simulink model "flightControlSystem"  (R2025b)
settings: Solver=ode3  StartTime=0  StopTime=TFinal  FixedStep=Ts  RelTol=1e-3  EnableMultiTasking=on
undefined symbols (not defined in the file): codertarget, Controller, DiscIntNeverNeededParam, Discrete, Estimator, g, gray, init, orient_ref, pos_ref, Sensors, Time, Ts, var_acc_angle_N, var_bias_gyr_N, var_gyro_p_N, Vehicle
libraries: simulink x40, slpidlib x5, ctrlSharedLib x4, sharedtransform x3, visiontextngfix x1, parrotlib x1
(part 3 of 3)

== matlab function flightControlSystem/Image Processing System/MATLAB Function ==
  data: var_yok input; binaryImg input; line_coords output; line_colors output; yaw_angle output; current_yaw input; length_90 output; on_track output; land_now output; detected output; target_offset output
function [line_coords, line_colors, yaw_angle, length_90, on_track,land_now,detected,target_offset] = pathFollower(var_yok, binaryImg, current_yaw)
% --- PARAMETRELER VE MATRİS HAZIRLIĞI ---
H = 90; W = 60; 
x0 = 30; y0 = 60;
angles = -15:5:195; % Bu 41 elemanlı bir dizidir
numAngles = length(angles); % Dinamik olarak 37 olur
maxLen = 200;
coder.extrinsic('imfindcircles');

% Matris boyutlarını 37 ışın + 2 güvenlik noktası = 39 yapıyoruz
line_coords = zeros(46,4);
line_colors = zeros(46,3); 

% Başlangıçta tüm çizgileri yeşil yap
for i = 1:45
    line_colors(i,:) = [0 250 0];
end

lengths = zeros(numAngles, 1);
on_track = 1; 

% --- 1. IŞINSAL (RAY-CASTING) TARAMA ---
for i = 1:numAngles
    theta = angles(i) * pi/180;
    r = 0;
    for k = 1:maxLen
        x = round(x0 + k*cos(theta));
        y = round(y0 - k*sin(theta));
        
        if x < 1 || x > W || y < 1 || y > H || binaryImg(y,x) == 0
            break;
        end
        r = k;
    end
    x_end = round(x0 + r*cos(theta));
    y_end = round(y0 - r*sin(theta));
    
    line_coords(i,:) = [x0 y0 x_end y_end];
    lengths(i) = r;
end

% Sağ (1. ışın) ve Sol (Sonuncu ışın) çizgilerini MOR yap
line_colors(1, :) = [160 32 240];   % Mor (Purple)
line_colors(numAngles, :) = [160 32 240]; 

% --- DİĞER HESAPLAMALAR ---
% En uzun 3 çizgiyi bul ve kırmızı yap (Eğer morlarla çakışmazsa)
[~, idx] = sort(lengths, 'descend');
top_idxs = idx(1:3);
for j = 1:3
    % Eğer en uzunlardan biri 0 veya 180 değilse kırmızı yap
    if top_idxs(j) ~= 1 && top_idxs(j) ~= numAngles
        line_colors(top_idxs(j), :) = [245 0 0];
    end
end

% 90 derece (Tam ön - 19. eleman) çizgisini mavi yap
line_colors(22, :) = [0 0 255]; 
length_90 = lengths(22);

% --- 2. GÜVENLİK KOLLARI VE ON_TRACK KONTROLÜ ---
offset_x = 6; offset_y = 18; 
right_x = max(1, min(W, round(x0 + offset_x)));
left_x  = max(1, min(W, round(x0 - offset_x)));
check_y = max(1, min(H, round(y0 - offset_y)));

if binaryImg(check_y, right_x) == 0 || binaryImg(check_y, left_x) == 0
    on_track = 0; 
end

% --- 3. YAW HESAPLAMA ---
if var_yok == 1
        w1 = lengths(top_idxs(1)); w2 = lengths(top_idxs(2)); w3 = lengths(top_idxs(3));
        avg_angle_deg = (angles(top_idxs(1))*w1 + angles(top_idxs(2))*w2 + angles(top_idxs(3))*w3) / (w1 + w2 + w3);
        error_yaw = (avg_angle_deg - 90) * pi/180;
        yaw_angle = current_yaw + (error_yaw);
else
    yaw_angle = current_yaw;
end

% --- 4. GÖRSELLEŞTİRME (38. ve 39. SATIRLAR) ---
line_coords(44,:) = [right_x, check_y, right_x+1, check_y];
line_coords(45,:) = [left_x, check_y, left_x+1, check_y];

% Güvenlik noktaları renkleri
if binaryImg(check_y, right_x) == 0
    line_colors(44,:) = [0 0 0]; 
else
    line_colors(44,:) = [255 255 255]; 
end

if binaryImg(check_y, left_x) == 0
    line_colors(45,:) = [0 0 0];
else
    line_colors(45,:) = [255 255 255];
end
%%%%%%%%%%%%%%%%%%%%%%%%%%%%%%%%%%%%%%%%%%%%%%%%%%%%%%
% Varsayılan değerler
center_out    = [0 0];
radii_out     = 0;
target_offset = [0; 0];
land_now      = 0;
detected = false;

[centers, radii] = imfindcircles(binaryImg, [10 50], 'Sensitivity', 0.78);
detected = ~isempty(centers);
% Eğer bir çember bulunduysa (isempty değilse) direkt ata
if ~isempty(centers)
    center_out = centers;    % Zaten tek bir satır (1x2) gelecek
    % Ofset hesaplama
    target_offset = (center_out - [x0 y0])';
    error_yaw = (atan(target_offset(2)/target_offset(1))*pi/180);
    yaw_angle = current_yaw + (error_yaw);
    
    % İniş koşulu
    if norm(target_offset) < 15
        land_now = 1;
    end
end
end

== matlab function flightControlSystem/Control System/Controller/Position Controller/Position error transformation (Earth to Body frame) ==
  data: yaw input; xy_err_earth input; xy_err_body output
function xy_err_body = fcn(yaw,xy_err_earth)

transformation = [cos(yaw), sin(yaw); -sin(yaw),  cos(yaw)];
xy_err_body = transformation * xy_err_earth;


end
